simulink library "RCD2"  (R2025b)
settings: Solver=VariableStepAuto  StartTime=0.0  StopTime=10.0  RelTol=1e-3
libraries: simulink x73, etargetslib x4, $bdroot x2
(part 1 of 2)
settings Model: Creator=Eisenblaetter  LastModifiedBy=Scythe
settings OptimizationCC: ReuseModelBlockBuffer=off
settings RTWCC: GPUComputeCapability=3.5

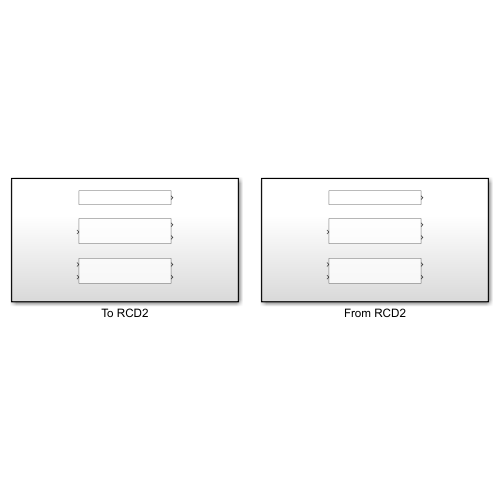
[thumbnail: Simulink's stored preview of the top-level diagram]
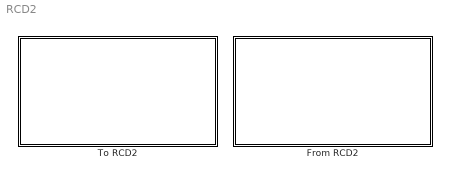
== system RCD2 ==
  From RCD2 : Subsystem
  To RCD2 : Subsystem

== system RCD2/From RCD2 ==
  RCD2 Actual Empty Bus : Subsystem
      mask help:
      | Create an empty RCD2 actual bus. All values are set to zero.<br><br>
      | The LED values are defined as follows:
      | <table style="background-color: #f8f8f8; border-style: solid; border-width: 1px; border-color: #ddd;" cellspacing="0" cellpadding ="2">
      | <tr style="background-color: #fff; text-align: left;"><th>Value</th><th>Description</th></tr>
      | <tr><td>0</td><td>LED off</td></tr>
      | <tr><td>1</td><td><span style="color: #f00;">RED</span> channel on, all others off</td></tr>
      | <tr><td>2</td><td><span style="color: #0f0;">GREEN</span> channel on, all others off</td></tr>
      | <tr><td>3</td><td><span style="color: #00f;">BLUE</span> channel on, all others off</td></tr>
      | </table>
      mask DialogControl DescGroupVar Prompt: RCD2 Actual - Empty Bus
      mask Display: disp('RCD2 Actual\nEmpty Bus');
  RCD2 Actual Pack : Subsystem  mask{idRCD=1}
      mask prompts: idRCD "ID of the RCD (0-255):"
      mask help:
      | Pack an RCD2 actual message to be sent from the RCD.<br><br>
      | The LED values are defined as follows:
      | <table style="background-color: #f8f8f8; border-style: solid; border-width: 1px; border-color: #ddd;" cellspacing="0" cellpadding ="2">
      | <tr style="background-color: #fff; text-align: left;"><th>Value</th><th>Description</th></tr>
      | <tr><td>0</td><td>LED off</td></tr>
      | <tr><td>1</td><td><span style="color: #f00;">RED</span> channel on, all others off</td></tr>
      | <tr><td>2</td><td><span style="color: #0f0;">GREEN</span> channel on, all others off</td></tr>
      | <tr><td>3</td><td><span style="color: #00f;">BLUE</span> channel on, all others off</td></tr>
      | </table>
      mask DialogControl DescGroupVar Prompt: RCD2 Actual - Pack
      mask Display:
      | id = get_param(gcb, 'idRCD');
      | disp(['RCD2 Actual\nPack\nID: ',id]);
  RCD2 Actual Unpack : Subsystem  mask{idRCD=1}
      mask prompts: idRCD "ID of the RCD (0-255):"
      mask help:
      | Pack an RCD2 actual message to be sent from the RCD.<br><br>
      | The LED values are defined as follows:
      | <table style="background-color: #f8f8f8; border-style: solid; border-width: 1px; border-color: #ddd;" cellspacing="0" cellpadding ="2">
      | <tr style="background-color: #fff; text-align: left;"><th>Value</th><th>Description</th></tr>
      | <tr><td>0</td><td>LED off</td></tr>
      | <tr><td>1</td><td><span style="color: #f00;">RED</span> channel on, all others off</td></tr>
      | <tr><td>2</td><td><span style="color: #0f0;">GREEN</span> channel on, all others off</td></tr>
      | <tr><td>3</td><td><span style="color: #00f;">BLUE</span> channel on, all others off</td></tr>
      | </table>
      mask DialogControl DescGroupVar Prompt: RCD2 Actual - Unpack
      mask Display:
      | id = get_param(gcb, 'idRCD');
      | disp(['RCD2 Actual\nUnpack\nID: ',id]);

== system RCD2/To RCD2 ==
  RCD2 Command Empty Bus : Subsystem
      mask help:
      | Create an empty RCD2 command bus. All values are set to zero and strings are empty.<br><br>
      | The LED values are defined as follows:
      | <table style="background-color: #f8f8f8; border-style: solid; border-width: 1px; border-color: #ddd;" cellspacing="0" cellpadding ="2">
      | <tr style="background-color: #fff; text-align: left;"><th>Value</th><th>Description</th></tr>
      | <tr><td>0</td><td>LED off</td></tr>
      | <tr><td>1</td><td><span style="color: #f00;">RED</span> channel on, all others off</td></tr>
      | <tr><td>2</td><td><span style="color: #0f0;">GREEN</span> channel on, all others off</td></tr>
      | <tr><td>3</td><td><span style="color: #00f;">BLUE</span> channel on, all others off</td></tr>
      | </table>
      mask DialogControl DescGroupVar Prompt: RCD2 Command - Empty Bus
      mask Display: disp('RCD2 Command\nEmpty Bus');
  RCD2 Command Pack : Subsystem  mask{idRCD=1}
      mask prompts: idRCD "ID of the RCD (0-255):"
      mask help:
      | Pack an RCD2 command message to be sent to the RCD.<br><br>
      | The LED values are defined as follows:
      | <table style="background-color: #f8f8f8; border-style: solid; border-width: 1px; border-color: #ddd;" cellspacing="0" cellpadding ="2">
      | <tr style="background-color: #fff; text-align: left;"><th>Value</th><th>Description</th></tr>
      | <tr><td>0</td><td>LED off</td></tr>
      | <tr><td>1</td><td><span style="color: #f00;">RED</span> channel on, all others off</td></tr>
      | <tr><td>2</td><td><span style="color: #0f0;">GREEN</span> channel on, all others off</td></tr>
      | <tr><td>3</td><td><span style="color: #00f;">BLUE</span> channel on, all others off</td></tr>
      | </table>
      mask DialogControl DescGroupVar Prompt: RCD2 Command - Pack
      mask Display:
      | id = get_param(gcb, 'idRCD');
      | disp(['RCD2 Command\nPack\nID: ',id]);
  RCD2 Command Unpack : Subsystem  mask{idRCD=1}
      mask prompts: idRCD "ID of the RCD (0-255):"
      mask help:
      | Unpack an RCD2 command message that has been sent to the RCD.<br><br>
      | The LED values are defined as follows:
      | <table style="background-color: #f8f8f8; border-style: solid; border-width: 1px; border-color: #ddd;" cellspacing="0" cellpadding ="2">
      | <tr style="background-color: #fff; text-align: left;"><th>Value</th><th>Description</th></tr>
      | <tr><td>0</td><td>LED off</td></tr>
      | <tr><td>1</td><td><span style="color: #f00;">RED</span> channel on, all others off</td></tr>
      | <tr><td>2</td><td><span style="color: #0f0;">GREEN</span> channel on, all others off</td></tr>
      | <tr><td>3</td><td><span style="color: #00f;">BLUE</span> channel on, all others off</td></tr>
      | </table>
      mask DialogControl DescGroupVar Prompt: RCD2 Command - Unpack
      mask Display:
      | id = get_param(gcb, 'idRCD');
      | disp(['RCD2 Command\nUnpack\nID: ',id]);

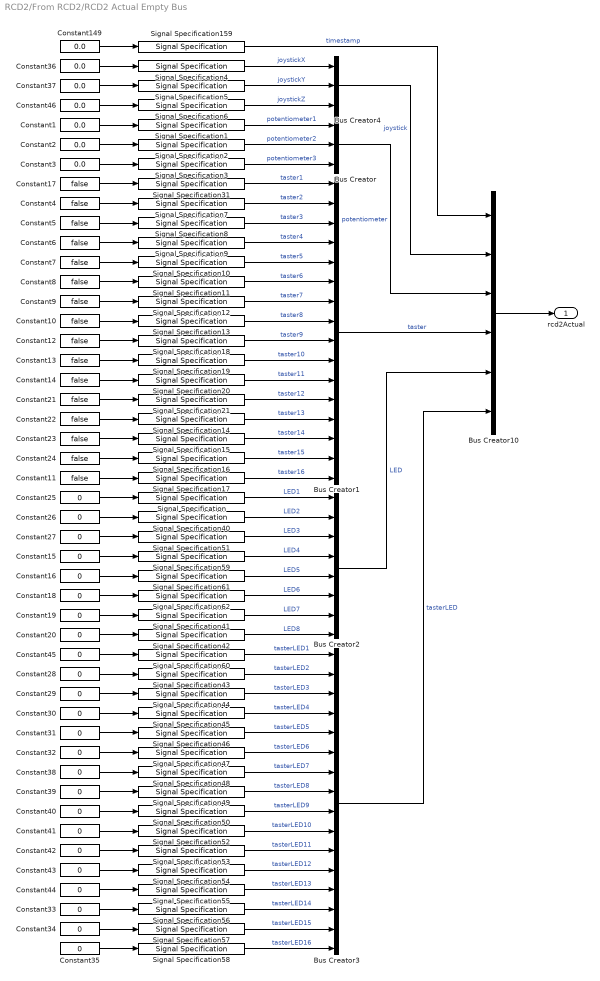
== system RCD2/From RCD2/RCD2 Actual Empty Bus ==
  Bus Creator : BusCreator  Inputs=3
  Bus Creator1 : BusCreator  Inputs=16
  Bus Creator10 : BusCreator  Inputs=6
  Bus Creator2 : BusCreator  Inputs=8
  Bus Creator3 : BusCreator  Inputs=16
  Bus Creator4 : BusCreator  Inputs=3
  Constant{1..3,36..37,46,149} (7 alike) : Constant  Value=0.0  OutDataTypeStr=double
  Constant{4..14,17,21..24} (16 alike) : Constant  Value=false  OutDataTypeStr=boolean
  Constant{15..16,18..20,25..35,38..45} (24 alike) : Constant  Value=0  OutDataTypeStr=uint8
  Signal Specification{,40..62} (24 alike) : SignalSpecification  OutDataTypeStr=uint8  Dimensions=1
  Signal Specification{1..6} (6 alike) : SignalSpecification  OutDataTypeStr=double  Dimensions=1
  Signal Specification{7..21,31} (16 alike) : SignalSpecification  OutDataTypeStr=boolean  Dimensions=1
  Signal Specification159 : SignalSpecification  OutDataTypeStr=double  Unit=s  Dimensions=1
  rcd2Actual : Outport
  wires:
  Bus Creator/1 -> Bus Creator10/3  "potentiometer"
  Signal Specification159/1 -> Bus Creator10/1  "timestamp"
  Bus Creator10/1 -> rcd2Actual/1
  Bus Creator1/1 -> Bus Creator10/4  "taster"
  Constant149/1 -> Signal Specification159/1
  Signal Specification53/1 -> Bus Creator3/11  "tasterLED11"
  Bus Creator2/1 -> Bus Creator10/5  "LED"
  Signal Specification55/1 -> Bus Creator3/13  "tasterLED13"
  Signal Specification43/1 -> Bus Creator3/2  "tasterLED2"
  Signal Specification50/1 -> Bus Creator3/9  "tasterLED9"
  Signal Specification51/1 -> Bus Creator2/3  "LED3"
  Signal Specification57/1 -> Bus Creator3/15  "tasterLED15"
  Signal Specification/1 -> Bus Creator2/1  "LED1"
  Signal Specification62/1 -> Bus Creator2/6  "LED6"
  Signal Specification59/1 -> Bus Creator2/4  "LED4"
  Bus Creator3/1 -> Bus Creator10/6  "tasterLED"
  Signal Specification49/1 -> Bus Creator3/8  "tasterLED8"
  Signal Specification44/1 -> Bus Creator3/3  "tasterLED3"
  Signal Specification40/1 -> Bus Creator2/2  "LED2"
  Signal Specification61/1 -> Bus Creator2/5  "LED5"
  Signal Specification45/1 -> Bus Creator3/4  "tasterLED4"
  Signal Specification42/1 -> Bus Creator2/8  "LED8"
  Signal Specification47/1 -> Bus Creator3/6  "tasterLED6"
  Signal Specification46/1 -> Bus Creator3/5  "tasterLED5"
  Signal Specification52/1 -> Bus Creator3/10  "tasterLED10"
  Signal Specification60/1 -> Bus Creator3/1  "tasterLED1"
  Signal Specification48/1 -> Bus Creator3/7  "tasterLED7"
  Signal Specification58/1 -> Bus Creator3/16  "tasterLED16"
  Signal Specification56/1 -> Bus Creator3/14  "tasterLED14"
  Signal Specification41/1 -> Bus Creator2/7  "LED7"
  Signal Specification54/1 -> Bus Creator3/12  "tasterLED12"
  Signal Specification21/1 -> Bus Creator1/12  "taster12"
  Signal Specification15/1 -> Bus Creator1/14  "taster14"
  Signal Specification17/1 -> Bus Creator1/16  "taster16"
  Constant17/1 -> Signal Specification31/1
  Signal Specification12/1 -> Bus Creator1/7  "taster7"
  Signal Specification31/1 -> Bus Creator1/1  "taster1"
  Signal Specification19/1 -> Bus Creator1/10  "taster10"
  Signal Specification10/1 -> Bus Creator1/5  "taster5"
  Signal Specification11/1 -> Bus Creator1/6  "taster6"
  Signal Specification9/1 -> Bus Creator1/4  "taster4"
  Signal Specification8/1 -> Bus Creator1/3  "taster3"
  Signal Specification13/1 -> Bus Creator1/8  "taster8"
  Signal Specification16/1 -> Bus Creator1/15  "taster15"
  Signal Specification18/1 -> Bus Creator1/9  "taster9"
  Signal Specification7/1 -> Bus Creator1/2  "taster2"
  Signal Specification14/1 -> Bus Creator1/13  "taster13"
  Signal Specification20/1 -> Bus Creator1/11  "taster11"
  Constant1/1 -> Signal Specification1/1
  Signal Specification1/1 -> Bus Creator/1  "potentiometer1"
  Constant2/1 -> Signal Specification2/1
  Signal Specification2/1 -> Bus Creator/2  "potentiometer2"
  Constant3/1 -> Signal Specification3/1
  Signal Specification3/1 -> Bus Creator/3  "potentiometer3"
  Constant27/1 -> Signal Specification51/1
  Constant15/1 -> Signal Specification59/1
  Constant16/1 -> Signal Specification61/1
  Constant20/1 -> Signal Specification42/1
  Constant19/1 -> Signal Specification41/1
  Constant18/1 -> Signal Specification62/1
  Constant25/1 -> Signal Specification/1
  Constant26/1 -> Signal Specification40/1
  Constant38/1 -> Signal Specification48/1
  Constant39/1 -> Signal Specification49/1
  Constant40/1 -> Signal Specification50/1
  Constant43/1 -> Signal Specification54/1
  Constant42/1 -> Signal Specification53/1
  Constant41/1 -> Signal Specification52/1
  Constant35/1 -> Signal Specification58/1
  Constant34/1 -> Signal Specification57/1
  Constant33/1 -> Signal Specification56/1
  Constant44/1 -> Signal Specification55/1
  Constant45/1 -> Signal Specification60/1
  Constant28/1 -> Signal Specification43/1
  Constant29/1 -> Signal Specification44/1
  Constant32/1 -> Signal Specification47/1
  Constant31/1 -> Signal Specification46/1
  Constant30/1 -> Signal Specification45/1
  Signal Specification6/1 -> Bus Creator4/3  "joystickZ"
  Constant46/1 -> Signal Specification6/1
  Signal Specification5/1 -> Bus Creator4/2  "joystickY"
  Constant37/1 -> Signal Specification5/1
  Signal Specification4/1 -> Bus Creator4/1  "joystickX"
  Constant36/1 -> Signal Specification4/1
  Bus Creator4/1 -> Bus Creator10/2  "joystick"
  Constant4/1 -> Signal Specification7/1
  Constant6/1 -> Signal Specification9/1
  Constant5/1 -> Signal Specification8/1
  Constant9/1 -> Signal Specification12/1
  Constant10/1 -> Signal Specification13/1
  Constant8/1 -> Signal Specification11/1
  Constant7/1 -> Signal Specification10/1
  Constant22/1 -> Signal Specification14/1
  Constant23/1 -> Signal Specification15/1
  Constant11/1 -> Signal Specification17/1
  Constant24/1 -> Signal Specification16/1
  Constant14/1 -> Signal Specification20/1
  Constant21/1 -> Signal Specification21/1
  Constant13/1 -> Signal Specification19/1
  Constant12/1 -> Signal Specification18/1

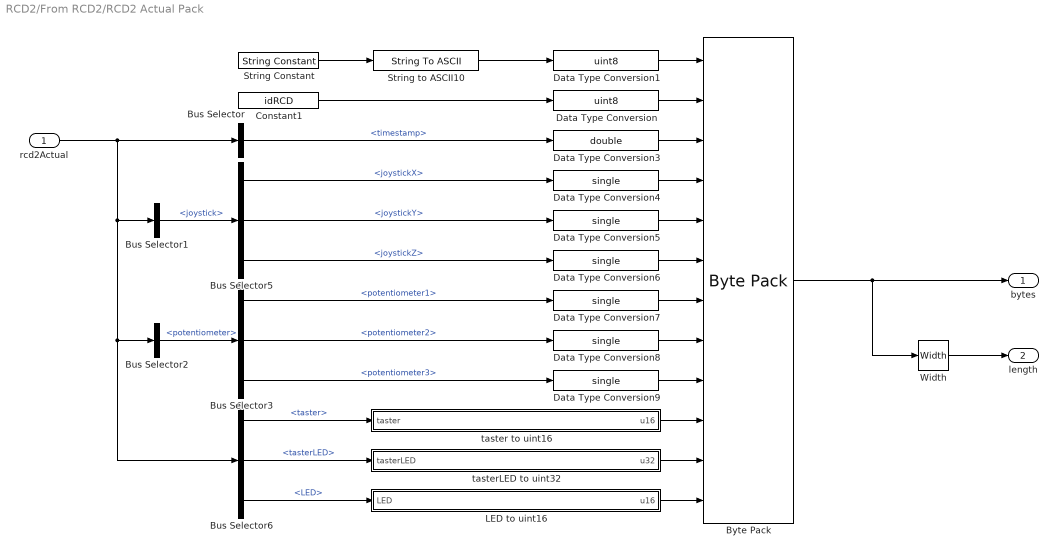
== system RCD2/From RCD2/RCD2 Actual Pack ==
  rcd2Actual : Inport
  Bus Selector : BusSelector  OutputSignals=timestamp
  Bus Selector1 : BusSelector  OutputSignals=joystick
  Bus Selector2 : BusSelector  OutputSignals=potentiometer
  Bus Selector3 : BusSelector  OutputSignals=potentiometer1,potentiometer2,potentiometer3
  Bus Selector5 : BusSelector  OutputSignals=joystickX,joystickY,joystickZ
  Bus Selector6 : BusSelector  OutputSignals=taster,tasterLED,LED
  Byte Pack : etargetslib/Byte Pack  datatypes={'uint8','uint8','double','single','single','single','single','single','single','uint16','uint32','uint16'}  byteAlign=1
  Constant1 : Constant  Value=idRCD  OutDataTypeStr=uint8
  Data Type Conversion : DataTypeConversion  OutDataTypeStr=uint8  SaturateOnIntegerOverflow=off  RndMeth=Floor
  Data Type Conversion1 : DataTypeConversion  OutDataTypeStr=uint8  SaturateOnIntegerOverflow=off  RndMeth=Floor
  Data Type Conversion3 : DataTypeConversion  OutDataTypeStr=double  SaturateOnIntegerOverflow=off  RndMeth=Floor
  Data Type Conversion{4..9} (6 alike) : DataTypeConversion  OutDataTypeStr=single  SaturateOnIntegerOverflow=off  RndMeth=Floor
  LED to uint16 : Subsystem
  String Constant : StringConstant  String="\"RCD2\""
  String to ASCII10 : StringToASCII  OutputVectorSize=4
  Width : Width  DataType=int32
  taster to uint16 : Subsystem
  tasterLED to uint32 : Subsystem
  bytes : Outport  OutDataTypeStr=uint8
  length : Outport  Port=2  OutDataTypeStr=int32  PortDimensions=1
  wires:
  Bus Selector5/1 -> Data Type Conversion4/1  "<joystickX>"
  Bus Selector5/2 -> Data Type Conversion5/1  "<joystickY>"
  Width/1 -> length/1
  Bus Selector5/3 -> Data Type Conversion6/1  "<joystickZ>"
  String Constant/1 -> String to ASCII10/1
  Constant1/1 -> Data Type Conversion/1
  String to ASCII10/1 -> Data Type Conversion1/1
  Bus Selector/1 -> Data Type Conversion3/1  "<timestamp>"
  Byte Pack/1 -> Width/1, bytes/1
  Bus Selector1/1 -> Bus Selector5/1  "<joystick>"
  Bus Selector2/1 -> Bus Selector3/1  "<potentiometer>"
  Bus Selector3/3 -> Data Type Conversion9/1  "<potentiometer3>"
  Bus Selector3/2 -> Data Type Conversion8/1  "<potentiometer2>"
  Bus Selector3/1 -> Data Type Conversion7/1  "<potentiometer1>"
  rcd2Actual/1 -> Bus Selector6/1, Bus Selector2/1, Bus Selector1/1, Bus Selector/1
  Bus Selector6/1 -> taster to uint16/1("taster ")  "<taster>"
  Bus Selector6/2 -> tasterLED to uint32/1("tasterLED ")  "<tasterLED>"
  Bus Selector6/3 -> LED to uint16/1("LED ")  "<LED>"
  Data Type Conversion6/1 -> Byte Pack/6
  Data Type Conversion7/1 -> Byte Pack/7
  Data Type Conversion8/1 -> Byte Pack/8
  Data Type Conversion9/1 -> Byte Pack/9
  taster to uint16/1(u16) -> Byte Pack/10
  tasterLED to uint32/1(u32) -> Byte Pack/11
  LED to uint16/1(u16) -> Byte Pack/12
  Data Type Conversion4/1 -> Byte Pack/4
  Data Type Conversion5/1 -> Byte Pack/5
  Data Type Conversion3/1 -> Byte Pack/3
  Data Type Conversion/1 -> Byte Pack/2
  Data Type Conversion1/1 -> Byte Pack/1

== system RCD2/From RCD2/RCD2 Actual Unpack ==
  bytes : Inport  OutDataTypeStr=uint8
  length : Inport  Port=2  OutDataTypeStr=int32  PortDimensions=1
  AND : Logic  AllPortsSameDT=off  OutDataTypeStr=boolean
  AND1 : Logic  AllPortsSameDT=off  OutDataTypeStr=boolean
  Check Message Size : simulink/Logic and Bit Operations/Compare To Constant  relop===  const=int32(45)  OutDataTypeStr=boolean
  Relational Operator : RelationalOperator  Operator=<=  OutDataTypeStr=boolean  RndMeth=Simplest  InputSameDT=off
  Unpack Message : Subsystem  TreatAsAtomicUnit=on
  Width : Width  DataType=int32
  success : Outport  OutDataTypeStr=boolean  PortDimensions=1
  rcd2Actual : Outport  Port=2
  wires:
  Unpack Message/1(success) -> AND/2
  Unpack Message/2(busRCDActual) -> rcd2Actual/1
  AND1/1 -> Unpack Message/Enable, AND/1
  AND/1 -> success/1
  Width/1 -> Relational Operator/2
  length/1 -> Relational Operator/1, Check Message Size/1
  Relational Operator/1 -> AND1/2
  bytes/1 -> Width/1, Unpack Message/1(bytes)
  Check Message Size/1 -> AND1/1

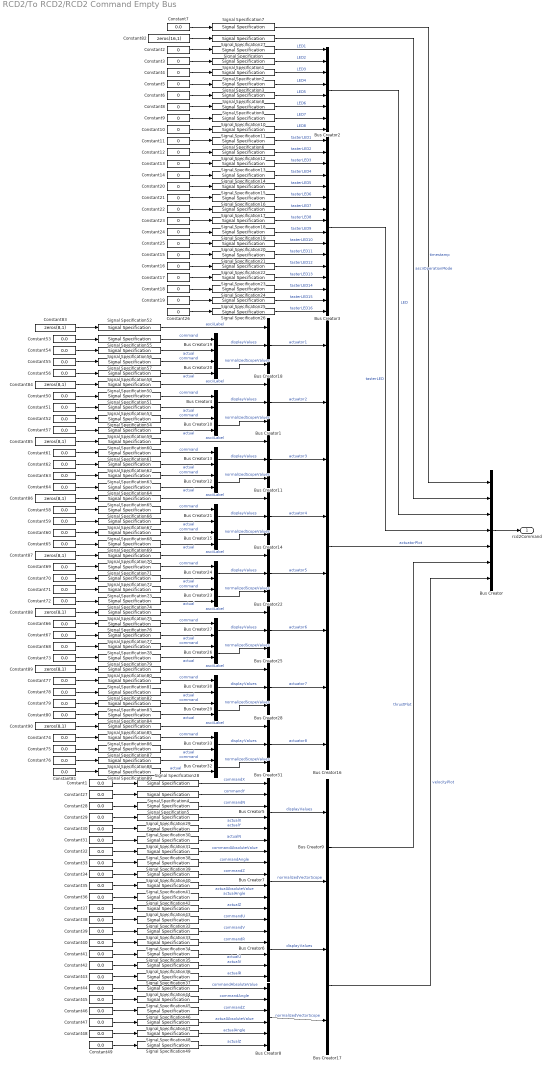
== system RCD2/To RCD2/RCD2 Command Empty Bus ==
  Bus Creator : BusCreator  Inputs=7
  Bus Creator{1,11,14,18,22,25,28,31} (8 alike) : BusCreator  Inputs=3
  Bus Creator{4,9..10,12..13,15,17,19..21,23..24,26..27,29..30,32..33} (18 alike) : BusCreator  Inputs=2
  Bus Creator16 : BusCreator  Inputs=8
  Bus Creator2 : BusCreator  Inputs=8
  Bus Creator3 : BusCreator  Inputs=16
  Bus Creator{5..8} (4 alike) : BusCreator  Inputs=6
  Constant{1,7,27..81} (57 alike) : Constant  Value=0.0  OutDataTypeStr=double
  Constant{2..6,8..26} (24 alike) : Constant  Value=0  OutDataTypeStr=uint8
  Constant82 : Constant  Value=zeros(16,1)  OutDataTypeStr=uint8
  Constant{83..90} (8 alike) : Constant  Value=zeros(8,1)  OutDataTypeStr=uint8
  Signal Specification{,1..3,6,8..26} (24 alike) : SignalSpecification  OutDataTypeStr=uint8  Dimensions=1
  Signal Specification27 : SignalSpecification  OutDataTypeStr=uint8  Dimensions=16
  Signal Specification{4..5,28..49,51,53..59,61..64,66..69,71..74,76..79,81..84,86..89} (56 alike) : SignalSpecification  OutDataTypeStr=double  Dimensions=1
  Signal Specification{50,52,60,65,70,75,80,85} (8 alike) : SignalSpecification  OutDataTypeStr=uint8  Dimensions=8
  Signal Specification7 : SignalSpecification  OutDataTypeStr=double  Unit=s  Dimensions=1
  rcd2Command : Outport
  wires:
  Bus Creator/1 -> rcd2Command/1
  Signal Specification22/1 -> Bus Creator3/12  "tasterLED12"
  Signal Specification5/1 -> Bus Creator5/3  "commandN"
  Constant39/1 -> Signal Specification33/1
  Constant29/1 -> Signal Specification29/1
  Bus Creator17/1 -> Bus Creator/7  "velocityPlot"
  Signal Specification23/1 -> Bus Creator3/13  "tasterLED13"
  Signal Specification2/1 -> Bus Creator2/3  "LED3"
  Signal Specification26/1 -> Bus Creator3/16  "tasterLED16"
  Constant82/1 -> Signal Specification27/1
  Constant15/1 -> Signal Specification21/1
  Constant7/1 -> Signal Specification7/1
  Constant2/1 -> Signal Specification/1
  Constant14/1 -> Signal Specification14/1
  Signal Specification16/1 -> Bus Creator3/6  "tasterLED6"
  Constant42/1 -> Signal Specification36/1
  Constant25/1 -> Signal Specification20/1
  Signal Specification30/1 -> Bus Creator5/5  "actualY"
  Bus Creator3/1 -> Bus Creator/4  "tasterLED"
  Bus Creator16/1 -> Bus Creator/5  "actuatorPlot"
  Signal Specification11/1 -> Bus Creator2/8  "LED8"
  Signal Specification17/1 -> Bus Creator3/7  "tasterLED7"
  Signal Specification29/1 -> Bus Creator5/4  "actualX"
  Constant28/1 -> Signal Specification5/1
  Constant12/1 -> Signal Specification12/1
  Constant31/1 -> Signal Specification31/1
  Signal Specification39/1 -> Bus Creator7/2  "commandAngle"
  Signal Specification10/1 -> Bus Creator2/7  "LED7"
  Signal Specification31/1 -> Bus Creator5/6  "actualN"
  Signal Specification1/1 -> Bus Creator2/2  "LED2"
  Signal Specification9/1 -> Bus Creator2/6  "LED6"
  Constant8/1 -> Signal Specification9/1
  Signal Specification4/1 -> Bus Creator5/2  "commandY"
  Constant17/1 -> Signal Specification23/1
  Bus Creator9/1 -> Bus Creator/6  "thrustPlot"
  Constant30/1 -> Signal Specification30/1
  Constant1/1 -> Signal Specification28/1
  Constant18/1 -> Signal Specification24/1
  Signal Specification35/1 -> Bus Creator6/4  "actualU"
  Constant5/1 -> Signal Specification3/1
  Signal Specification36/1 -> Bus Creator6/5  "actualV"
  Constant32/1 -> Signal Specification38/1
  Signal Specification14/1 -> Bus Creator3/4  "tasterLED4"
  Signal Specification21/1 -> Bus Creator3/11  "tasterLED11"
  Signal Specification42/1 -> Bus Creator7/5  "actualAngle"
  Signal Specification13/1 -> Bus Creator3/3  "tasterLED3"
  Bus Creator2/1 -> Bus Creator/3  "LED"
  Constant41/1 -> Signal Specification35/1
  Constant40/1 -> Signal Specification34/1
  Constant34/1 -> Signal Specification40/1
  Constant38/1 -> Signal Specification32/1
  Signal Specification34/1 -> Bus Creator6/3  "commandR"
  Constant27/1 -> Signal Specification4/1
  Signal Specification32/1 -> Bus Creator6/1  "commandU"
  Signal Specification28/1 -> Bus Creator5/1  "commandX"
  Signal Specification33/1 -> Bus Creator6/2  "commandV"
  Signal Specification40/1 -> Bus Creator7/3  "commandZ"
  Signal Specification/1 -> Bus Creator2/1  "LED1"
  Constant43/1 -> Signal Specification37/1
  Constant26/1 -> Signal Specification26/1
  Constant37/1 -> Signal Specification43/1
  Constant35/1 -> Signal Specification41/1
  Signal Specification20/1 -> Bus Creator3/10  "tasterLED10"
  Signal Specification38/1 -> Bus Creator7/1  "commandAbsoluteValue"
  Constant3/1 -> Signal Specification1/1
  Constant36/1 -> Signal Specification42/1
  Signal Specification3/1 -> Bus Creator2/4  "LED4"
  Signal Specification24/1 -> Bus Creator3/14  "tasterLED14"
  Constant16/1 -> Signal Specification22/1
  Constant19/1 -> Signal Specification25/1
  Signal Specification12/1 -> Bus Creator3/2  "tasterLED2"
  Constant20/1 -> Signal Specification15/1
  Constant11/1 -> Signal Specification6/1
  Constant9/1 -> Signal Specification10/1
  Signal Specification43/1 -> Bus Creator7/6  "actualZ"
  Constant10/1 -> Signal Specification11/1
  Signal Specification19/1 -> Bus Creator3/9  "tasterLED9"
  Constant6/1 -> Signal Specification8/1
  Constant21/1 -> Signal Specification16/1
  Signal Specification15/1 -> Bus Creator3/5  "tasterLED5"
  Signal Specification25/1 -> Bus Creator3/15  "tasterLED15"
  Constant33/1 -> Signal Specification39/1
  Constant13/1 -> Signal Specification13/1
  Signal Specification37/1 -> Bus Creator6/6  "actualR"
  Signal Specification18/1 -> Bus Creator3/8  "tasterLED8"
  Signal Specification8/1 -> Bus Creator2/5  "LED5"
  Signal Specification41/1 -> Bus Creator7/4  "actualAbsoluteValue"
  Constant23/1 -> Signal Specification18/1
  Constant24/1 -> Signal Specification19/1
  Constant4/1 -> Signal Specification2/1
  Signal Specification6/1 -> Bus Creator3/1  "tasterLED1"
  Signal Specification7/1 -> Bus Creator/1  "timestamp"
  Constant22/1 -> Signal Specification17/1
  Signal Specification27/1 -> Bus Creator/2  "asciiOperationMode"
  Signal Specification47/1 -> Bus Creator8/4  "actualAbsoluteValue"
  Constant45/1 -> Signal Specification45/1
  Signal Specification49/1 -> Bus Creator8/6  "actualZ"
  Constant48/1 -> Signal Specification48/1
  Signal Specification44/1 -> Bus Creator8/1  "commandAbsoluteValue"
  Constant47/1 -> Signal Specification47/1
  Constant49/1 -> Signal Specification49/1
  Signal Specification46/1 -> Bus Creator8/3  "commandZ"
  Constant46/1 -> Signal Specification46/1
  Signal Specification48/1 -> Bus Creator8/5  "actualAngle"
  Constant44/1 -> Signal Specification44/1
  Signal Specification45/1 -> Bus Creator8/2  "commandAngle"
  Bus Creator11/1 -> Bus Creator16/3  "actuator3"
  Bus Creator14/1 -> Bus Creator16/4  "actuator4"
  Bus Creator1/1 -> Bus Creator16/2  "actuator2"
  Bus Creator22/1 -> Bus Creator16/5  "actuator5"
  Bus Creator18/1 -> Bus Creator16/1  "actuator1"
  Bus Creator25/1 -> Bus Creator16/6  "actuator6"
  Bus Creator28/1 -> Bus Creator16/7  "actuator7"
  Bus Creator31/1 -> Bus Creator16/8  "actuator8"
  Bus Creator5/1 -> Bus Creator9/1  "displayValues"
  Bus Creator7/1 -> Bus Creator9/2  "normalizedVectorScope"
  Bus Creator6/1 -> Bus Creator17/1  "displayValues"
  Bus Creator8/1 -> Bus Creator17/2  "normalizedVectorScope"
  Constant54/1 -> Signal Specification56/1
  Constant53/1 -> Signal Specification55/1
  Signal Specification56/1 -> Bus Creator19/2  "actual"
  Signal Specification52/1 -> Bus Creator18/1  "asciiLabel"
  Constant83/1 -> Signal Specification52/1
  Signal Specification55/1 -> Bus Creator19/1  "command"
  Bus Creator19/1 -> Bus Creator18/2  "displayValues"
  Bus Creator20/1 -> Bus Creator18/3  "normalizedScopeValues"
  Signal Specification57/1 -> Bus Creator20/1  "command"
  Signal Specification58/1 -> Bus Creator20/2  "actual"
  Constant55/1 -> Signal Specification57/1
  Constant56/1 -> Signal Specification58/1
  Constant57/1 -> Signal Specification59/1
  Constant52/1 -> Signal Specification54/1
  Signal Specification59/1 -> Bus Creator10/2  "actual"
  Signal Specification54/1 -> Bus Creator10/1  "command"
  Bus Creator10/1 -> Bus Creator1/3  "normalizedScopeValues"
  Bus Creator4/1 -> Bus Creator1/2  "displayValues"
  Signal Specification51/1 -> Bus Creator4/1  "command"
  Signal Specification53/1 -> Bus Creator4/2  "actual"
  Constant50/1 -> Signal Specification51/1
  Constant51/1 -> Signal Specification53/1
  Constant62/1 -> Signal Specification62/1
  Constant61/1 -> Signal Specification61/1
  Signal Specification62/1 -> Bus Creator13/2  "actual"
  Signal Specification61/1 -> Bus Creator13/1  "command"
  Bus Creator13/1 -> Bus Creator11/2  "displayValues"
  Bus Creator12/1 -> Bus Creator11/3  "normalizedScopeValues"
  Signal Specification63/1 -> Bus Creator12/1  "command"
  Signal Specification64/1 -> Bus Creator12/2  "actual"
  Constant63/1 -> Signal Specification63/1
  Constant64/1 -> Signal Specification64/1
  Constant65/1 -> Signal Specification69/1
  Constant60/1 -> Signal Specification68/1
  Signal Specification69/1 -> Bus Creator15/2  "actual"
  Signal Specification68/1 -> Bus Creator15/1  "command"
  Bus Creator15/1 -> Bus Creator14/3  "normalizedScopeValues"
  Bus Creator21/1 -> Bus Creator14/2  "displayValues"
  Signal Specification66/1 -> Bus Creator21/1  "command"
  Signal Specification67/1 -> Bus Creator21/2  "actual"
  Constant58/1 -> Signal Specification66/1
  Constant59/1 -> Signal Specification67/1
  Constant70/1 -> Signal Specification72/1
  Constant69/1 -> Signal Specification71/1
  Signal Specification72/1 -> Bus Creator24/2  "actual"
  Signal Specification71/1 -> Bus Creator24/1  "command"
  Bus Creator24/1 -> Bus Creator22/2  "displayValues"
  Bus Creator23/1 -> Bus Creator22/3  "normalizedScopeValues"
  Signal Specification73/1 -> Bus Creator23/1  "command"
  Signal Specification74/1 -> Bus Creator23/2  "actual"
  Constant71/1 -> Signal Specification73/1
  Constant72/1 -> Signal Specification74/1
  Constant73/1 -> Signal Specification79/1
  Constant68/1 -> Signal Specification78/1
  Signal Specification79/1 -> Bus Creator26/2  "actual"
  Signal Specification78/1 -> Bus Creator26/1  "command"
  Bus Creator26/1 -> Bus Creator25/3  "normalizedScopeValues"
  Bus Creator27/1 -> Bus Creator25/2  "displayValues"
  Signal Specification76/1 -> Bus Creator27/1  "command"
  Signal Specification77/1 -> Bus Creator27/2  "actual"
  Constant66/1 -> Signal Specification76/1
  Constant67/1 -> Signal Specification77/1
  Constant78/1 -> Signal Specification82/1
  Constant77/1 -> Signal Specification81/1
  Signal Specification82/1 -> Bus Creator30/2  "actual"
  Signal Specification81/1 -> Bus Creator30/1  "command"
  Bus Creator30/1 -> Bus Creator28/2  "displayValues"
  Bus Creator29/1 -> Bus Creator28/3  "normalizedScopeValues"
  Signal Specification83/1 -> Bus Creator29/1  "command"
  Signal Specification84/1 -> Bus Creator29/2  "actual"
  Constant79/1 -> Signal Specification83/1
  Constant80/1 -> Signal Specification84/1
  Constant81/1 -> Signal Specification89/1
  Constant76/1 -> Signal Specification88/1
  Signal Specification89/1 -> Bus Creator32/2  "actual"
  Signal Specification88/1 -> Bus Creator32/1  "command"
  Bus Creator32/1 -> Bus Creator31/3  "normalizedScopeValues"
  Bus Creator33/1 -> Bus Creator31/2  "displayValues"
  Signal Specification86/1 -> Bus Creator33/1  "command"
  Signal Specification87/1 -> Bus Creator33/2  "actual"
  Constant74/1 -> Signal Specification86/1
  Constant75/1 -> Signal Specification87/1
  Signal Specification50/1 -> Bus Creator1/1  "asciiLabel"
  Signal Specification60/1 -> Bus Creator11/1  "asciiLabel"
  Signal Specification65/1 -> Bus Creator14/1  "asciiLabel"
  Signal Specification70/1 -> Bus Creator22/1  "asciiLabel"
  Signal Specification75/1 -> Bus Creator25/1  "asciiLabel"
  Signal Specification80/1 -> Bus Creator28/1  "asciiLabel"
  Signal Specification85/1 -> Bus Creator31/1  "asciiLabel"
  Constant84/1 -> Signal Specification50/1
  Constant85/1 -> Signal Specification60/1
  Constant86/1 -> Signal Specification65/1
  Constant87/1 -> Signal Specification70/1
  Constant88/1 -> Signal Specification75/1
  Constant89/1 -> Signal Specification80/1
  Constant90/1 -> Signal Specification85/1

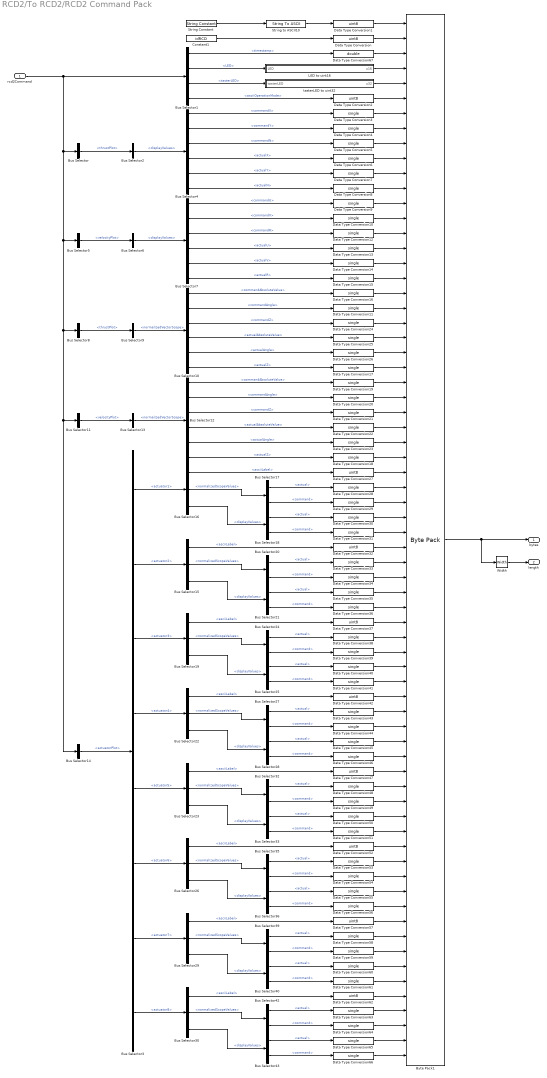
== system RCD2/To RCD2/RCD2 Command Pack ==
  rcd2Command : Inport
  Bus Selector : BusSelector  OutputSignals=thrustPlot
  Bus Selector1 : BusSelector  OutputSignals=timestamp,LED,tasterLED,asciiOperationMode
  Bus Selector10 : BusSelector  OutputSignals=commandAbsoluteValue,commandAngle,commandZ,actualAbsoluteValue,actualAngle,actualZ
  Bus Selector11 : BusSelector  OutputSignals=velocityPlot
  Bus Selector12 : BusSelector  OutputSignals=commandAbsoluteValue,commandAngle,commandZ,actualAbsoluteValue,actualAngle,actualZ
  Bus Selector13 : BusSelector  OutputSignals=normalizedVectorScope
  Bus Selector14 : BusSelector  OutputSignals=actuatorPlot
  Bus Selector{15..16,19,22..23,26,29..30} (8 alike) : BusSelector  OutputSignals=asciiLabel,normalizedScopeValues,displayValues
  Bus Selector{17..18,20..21,24..25,27..28,32..33,35..36,39..40,42..43} (16 alike) : BusSelector  OutputSignals=actual,command
  Bus Selector2 : BusSelector  OutputSignals=displayValues
  Bus Selector3 : BusSelector  OutputSignals=actuator1,actuator2,actuator3,actuator4,actuator5,actuator6,actuator7,actuator8
  Bus Selector4 : BusSelector  OutputSignals=commandX,commandY,commandN,actualX,actualY,actualN
  Bus Selector5 : BusSelector  OutputSignals=velocityPlot
  Bus Selector6 : BusSelector  OutputSignals=displayValues
  Bus Selector7 : BusSelector  OutputSignals=commandU,commandV,commandR,actualU,actualV,actualR
  Bus Selector8 : BusSelector  OutputSignals=thrustPlot
  Bus Selector9 : BusSelector  OutputSignals=normalizedVectorScope
  Byte Pack1 : etargetslib/Byte Pack  datatypes={'uint8', 'uint8', 'double', 'uint16','uint32','uint8','single','single','single','single','single','single','single','single','single','single','single','single','single','single','single','single','single','single','single','single','single','single','single','single','uint8','single','single','single','single','uint8','single','single','single','single','uint8','single','single','single','single','uint8','single','single','single','single','uint8','single','single','single','single','uint8','single','single','single','single','uint8','single','single','single','single','uint8','single','single','single','single'}  byteAlign=1
  Constant1 : Constant  Value=idRCD  OutDataTypeStr=uint8
  Data Type Conversion{,1..2,27,32,37,42,47,52,57,62} (11 alike) : DataTypeConversion  OutDataTypeStr=uint8  SaturateOnIntegerOverflow=off  RndMeth=Floor
  Data Type Conversion{3..26,28..31,33..36,38..41,43..46,48..51,53..56,58..61,63..66} (56 alike) : DataTypeConversion  OutDataTypeStr=single  SaturateOnIntegerOverflow=off  RndMeth=Floor
  Data Type Conversion67 : DataTypeConversion  OutDataTypeStr=double  SaturateOnIntegerOverflow=off  RndMeth=Floor
  LED to uint16 : Subsystem
  String Constant : StringConstant  String="\"RCD2\""
  String to ASCII10 : StringToASCII  OutputVectorSize=4
  Width : Width  DataType=int32
  tasterLED to uint32 : Subsystem
  bytes : Outport  OutDataTypeStr=uint8
  length : Outport  Port=2  OutDataTypeStr=int32  PortDimensions=1
  wires:
  Bus Selector1/3 -> tasterLED to uint32/1("tasterLED ")  "<tasterLED>"
  String to ASCII10/1 -> Data Type Conversion1/1
  Bus Selector1/2 -> LED to uint16/1("LED ")  "<LED>"
  Bus Selector1/4 -> Data Type Conversion2/1  "<asciiOperationMode>"
  String Constant/1 -> String to ASCII10/1
  tasterLED to uint32/1(u32) -> Byte Pack1/5
  Bus Selector1/1 -> Data Type Conversion67/1  "<timestamp>"
  LED to uint16/1(u16) -> Byte Pack1/4
  Data Type Conversion/1 -> Byte Pack1/2
  Byte Pack1/1 -> Width/1, bytes/1
  Width/1 -> length/1
  Constant1/1 -> Data Type Conversion/1
  Data Type Conversion1/1 -> Byte Pack1/1
  Data Type Conversion2/1 -> Byte Pack1/6
  Data Type Conversion3/1 -> Byte Pack1/7
  Data Type Conversion4/1 -> Byte Pack1/8
  Data Type Conversion5/1 -> Byte Pack1/9
  Data Type Conversion6/1 -> Byte Pack1/10
  Data Type Conversion7/1 -> Byte Pack1/11
  Data Type Conversion8/1 -> Byte Pack1/12
  Data Type Conversion9/1 -> Byte Pack1/13
  Data Type Conversion10/1 -> Byte Pack1/14
  Data Type Conversion12/1 -> Byte Pack1/15
  Data Type Conversion13/1 -> Byte Pack1/16
  Data Type Conversion14/1 -> Byte Pack1/17
  Data Type Conversion15/1 -> Byte Pack1/18
  Data Type Conversion16/1 -> Byte Pack1/19
  Data Type Conversion11/1 -> Byte Pack1/20
  Data Type Conversion24/1 -> Byte Pack1/21
  Data Type Conversion25/1 -> Byte Pack1/22
  Data Type Conversion26/1 -> Byte Pack1/23
  Data Type Conversion17/1 -> Byte Pack1/24
  Data Type Conversion19/1 -> Byte Pack1/25
  Data Type Conversion20/1 -> Byte Pack1/26
  Data Type Conversion21/1 -> Byte Pack1/27
  Data Type Conversion22/1 -> Byte Pack1/28
  Data Type Conversion23/1 -> Byte Pack1/29
  Data Type Conversion18/1 -> Byte Pack1/30
  Bus Selector/1 -> Bus Selector2/1  "<thrustPlot>"
  Bus Selector2/1 -> Bus Selector4/1  "<displayValues>"
  Bus Selector4/1 -> Data Type Conversion3/1  "<commandX>"
  Bus Selector4/2 -> Data Type Conversion4/1  "<commandY>"
  Bus Selector4/3 -> Data Type Conversion5/1  "<commandN>"
  Bus Selector4/4 -> Data Type Conversion6/1  "<actualX>"
  Bus Selector4/5 -> Data Type Conversion7/1  "<actualY>"
  Bus Selector4/6 -> Data Type Conversion8/1  "<actualN>"
  Bus Selector7/6 -> Data Type Conversion15/1  "<actualR>"
  Bus Selector7/5 -> Data Type Conversion14/1  "<actualV>"
  Bus Selector7/4 -> Data Type Conversion13/1  "<actualU>"
  Bus Selector7/3 -> Data Type Conversion12/1  "<commandR>"
  Bus Selector7/2 -> Data Type Conversion10/1  "<commandV>"
  Bus Selector7/1 -> Data Type Conversion9/1  "<commandU>"
  Bus Selector6/1 -> Bus Selector7/1  "<displayValues>"
  Bus Selector5/1 -> Bus Selector6/1  "<velocityPlot>"
  Bus Selector8/1 -> Bus Selector9/1  "<thrustPlot>"
  Bus Selector9/1 -> Bus Selector10/1  "<normalizedVectorScope>"
  Bus Selector10/1 -> Data Type Conversion16/1  "<commandAbsoluteValue>"
  Bus Selector10/2 -> Data Type Conversion11/1  "<commandAngle>"
  Bus Selector10/3 -> Data Type Conversion24/1  "<commandZ>"
  Bus Selector10/4 -> Data Type Conversion25/1  "<actualAbsoluteValue>"
  Bus Selector10/5 -> Data Type Conversion26/1  "<actualAngle>"
  Bus Selector10/6 -> Data Type Conversion17/1  "<actualZ>"
  Bus Selector12/6 -> Data Type Conversion18/1  "<actualZ>"
  Bus Selector12/5 -> Data Type Conversion23/1  "<actualAngle>"
  Bus Selector12/4 -> Data Type Conversion22/1  "<actualAbsoluteValue>"
  Bus Selector12/3 -> Data Type Conversion21/1  "<commandZ>"
  Bus Selector12/2 -> Data Type Conversion20/1  "<commandAngle>"
  Bus Selector12/1 -> Data Type Conversion19/1  "<commandAbsoluteValue>"
  Bus Selector13/1 -> Bus Selector12/1  "<normalizedVectorScope>"
  Bus Selector11/1 -> Bus Selector13/1  "<velocityPlot>"
  rcd2Command/1 -> Bus Selector14/1, Bus Selector11/1, Bus Selector8/1, Bus Selector5/1, Bus Selector/1, Bus Selector1/1
  Data Type Conversion27/1 -> Byte Pack1/31
  Bus Selector16/1 -> Data Type Conversion27/1  "<asciiLabel>"
  Bus Selector16/2 -> Bus Selector17/1  "<normalizedScopeValues>"
  Data Type Conversion28/1 -> Byte Pack1/32
  Data Type Conversion29/1 -> Byte Pack1/33
  Bus Selector17/1 -> Data Type Conversion28/1  "<actual>"
  Bus Selector17/2 -> Data Type Conversion29/1  "<command>"
  Bus Selector18/2 -> Data Type Conversion31/1  "<command>"
  Bus Selector18/1 -> Data Type Conversion30/1  "<actual>"
  Bus Selector16/3 -> Bus Selector18/1  "<displayValues>"
  Data Type Conversion30/1 -> Byte Pack1/34
  Data Type Conversion31/1 -> Byte Pack1/35
  Data Type Conversion36/1 -> Byte Pack1/40
  Data Type Conversion35/1 -> Byte Pack1/39
  Bus Selector15/3 -> Bus Selector21/1  "<displayValues>"
  Bus Selector21/1 -> Data Type Conversion35/1  "<actual>"
  Bus Selector21/2 -> Data Type Conversion36/1  "<command>"
  Bus Selector20/2 -> Data Type Conversion34/1  "<command>"
  Bus Selector20/1 -> Data Type Conversion33/1  "<actual>"
  Data Type Conversion34/1 -> Byte Pack1/38
  Data Type Conversion33/1 -> Byte Pack1/37
  Bus Selector15/2 -> Bus Selector20/1  "<normalizedScopeValues>"
  Bus Selector15/1 -> Data Type Conversion32/1  "<asciiLabel>"
  Data Type Conversion32/1 -> Byte Pack1/36
  Data Type Conversion42/1 -> Byte Pack1/46
  Bus Selector22/1 -> Data Type Conversion42/1  "<asciiLabel>"
  Bus Selector22/2 -> Bus Selector27/1  "<normalizedScopeValues>"
  Data Type Conversion43/1 -> Byte Pack1/47
  Data Type Conversion44/1 -> Byte Pack1/48
  Bus Selector27/1 -> Data Type Conversion43/1  "<actual>"
  Bus Selector27/2 -> Data Type Conversion44/1  "<command>"
  Bus Selector28/2 -> Data Type Conversion46/1  "<command>"
  Bus Selector28/1 -> Data Type Conversion45/1  "<actual>"
  Bus Selector22/3 -> Bus Selector28/1  "<displayValues>"
  Data Type Conversion45/1 -> Byte Pack1/49
  Data Type Conversion46/1 -> Byte Pack1/50
  Data Type Conversion41/1 -> Byte Pack1/45
  Data Type Conversion40/1 -> Byte Pack1/44
  Bus Selector19/3 -> Bus Selector25/1  "<displayValues>"
  Bus Selector25/1 -> Data Type Conversion40/1  "<actual>"
  Bus Selector25/2 -> Data Type Conversion41/1  "<command>"
  Bus Selector24/2 -> Data Type Conversion39/1  "<command>"
  Bus Selector24/1 -> Data Type Conversion38/1  "<actual>"
  Data Type Conversion39/1 -> Byte Pack1/43
  Data Type Conversion38/1 -> Byte Pack1/42
  Bus Selector19/2 -> Bus Selector24/1  "<normalizedScopeValues>"
  Bus Selector19/1 -> Data Type Conversion37/1  "<asciiLabel>"
  Data Type Conversion37/1 -> Byte Pack1/41
  Data Type Conversion57/1 -> Byte Pack1/61
  Bus Selector29/1 -> Data Type Conversion57/1  "<asciiLabel>"
  Bus Selector29/2 -> Bus Selector39/1  "<normalizedScopeValues>"
  Data Type Conversion58/1 -> Byte Pack1/62
  Data Type Conversion59/1 -> Byte Pack1/63
  Bus Selector39/1 -> Data Type Conversion58/1  "<actual>"
  Bus Selector39/2 -> Data Type Conversion59/1  "<command>"
  Bus Selector40/2 -> Data Type Conversion61/1  "<command>"
  Bus Selector40/1 -> Data Type Conversion60/1  "<actual>"
  Bus Selector29/3 -> Bus Selector40/1  "<displayValues>"
  Data Type Conversion60/1 -> Byte Pack1/64
  Data Type Conversion61/1 -> Byte Pack1/65
  Data Type Conversion66/1 -> Byte Pack1/70
  Data Type Conversion65/1 -> Byte Pack1/69
  Bus Selector30/3 -> Bus Selector43/1  "<displayValues>"
  Bus Selector43/1 -> Data Type Conversion65/1  "<actual>"
  Bus Selector43/2 -> Data Type Conversion66/1  "<command>"
  Bus Selector42/2 -> Data Type Conversion64/1  "<command>"
  Bus Selector42/1 -> Data Type Conversion63/1  "<actual>"
  Data Type Conversion64/1 -> Byte Pack1/68
  Data Type Conversion63/1 -> Byte Pack1/67
  Bus Selector30/2 -> Bus Selector42/1  "<normalizedScopeValues>"
  Bus Selector30/1 -> Data Type Conversion62/1  "<asciiLabel>"
  Data Type Conversion62/1 -> Byte Pack1/66
  Data Type Conversion52/1 -> Byte Pack1/56
  Bus Selector26/1 -> Data Type Conversion52/1  "<asciiLabel>"
  Bus Selector26/2 -> Bus Selector35/1  "<normalizedScopeValues>"
  Data Type Conversion53/1 -> Byte Pack1/57
  Data Type Conversion54/1 -> Byte Pack1/58
  Bus Selector35/1 -> Data Type Conversion53/1  "<actual>"
  Bus Selector35/2 -> Data Type Conversion54/1  "<command>"
  Bus Selector36/2 -> Data Type Conversion56/1  "<command>"
  Bus Selector36/1 -> Data Type Conversion55/1  "<actual>"
  Bus Selector26/3 -> Bus Selector36/1  "<displayValues>"
  Data Type Conversion55/1 -> Byte Pack1/59
  Data Type Conversion56/1 -> Byte Pack1/60
  Data Type Conversion51/1 -> Byte Pack1/55
  Data Type Conversion50/1 -> Byte Pack1/54
  Bus Selector23/3 -> Bus Selector33/1  "<displayValues>"
  Bus Selector33/1 -> Data Type Conversion50/1  "<actual>"
  Bus Selector33/2 -> Data Type Conversion51/1  "<command>"
  Bus Selector32/2 -> Data Type Conversion49/1  "<command>"
  Bus Selector32/1 -> Data Type Conversion48/1  "<actual>"
  Data Type Conversion49/1 -> Byte Pack1/53
  Data Type Conversion48/1 -> Byte Pack1/52
  Bus Selector23/2 -> Bus Selector32/1  "<normalizedScopeValues>"
  Bus Selector23/1 -> Data Type Conversion47/1  "<asciiLabel>"
  Data Type Conversion47/1 -> Byte Pack1/51
  Bus Selector14/1 -> Bus Selector3/1  "<actuatorPlot>"
  Bus Selector3/5 -> Bus Selector23/1  "<actuator5>"
  Bus Selector3/4 -> Bus Selector22/1  "<actuator4>"
  Bus Selector3/6 -> Bus Selector26/1  "<actuator6>"
  Bus Selector3/3 -> Bus Selector19/1  "<actuator3>"
  Bus Selector3/7 -> Bus Selector29/1  "<actuator7>"
  Bus Selector3/2 -> Bus Selector15/1  "<actuator2>"
  Bus Selector3/8 -> Bus Selector30/1  "<actuator8>"
  Bus Selector3/1 -> Bus Selector16/1  "<actuator1>"
  Data Type Conversion67/1 -> Byte Pack1/3

== system RCD2/To RCD2/RCD2 Command Unpack ==
  bytes : Inport  OutDataTypeStr=uint8
  length : Inport  Port=2  OutDataTypeStr=int32  PortDimensions=1
  AND : Logic  AllPortsSameDT=off  OutDataTypeStr=boolean
  AND1 : Logic  AllPortsSameDT=off  OutDataTypeStr=boolean
  Check Message Size : simulink/Logic and Bit Operations/Compare To Constant  relop===  const=int32(323)  OutDataTypeStr=boolean
  Relational Operator : RelationalOperator  Operator=<=  OutDataTypeStr=boolean  RndMeth=Simplest  InputSameDT=off
  Unpack Message : Subsystem  TreatAsAtomicUnit=on
  Width : Width  DataType=int32
  success : Outport
  rcd2Command : Outport  Port=2
  wires:
  bytes/1 -> Width/1, Unpack Message/1(bytes)
  AND1/1 -> Unpack Message/Enable, AND/1
  AND/1 -> success/1
  length/1 -> Relational Operator/1, Check Message Size/1
  Unpack Message/1(success) -> AND/2
  Unpack Message/2(busRCDCommand) -> rcd2Command/1
  Check Message Size/1 -> AND1/1
  Relational Operator/1 -> AND1/2
  Width/1 -> Relational Operator/2

== system RCD2/From RCD2/RCD2 Actual Pack/LED to uint16 ==
  "LED " : Inport
  Bitwise AND5 : simulink/Logic and Bit Operations/Bitwise Operator  logicop=OR  UseBitMask=off  NumInputPorts=8  BitMask=bin2dec('11011001')  BitMaskRealWorld=Stored Integer
      settings: LibrarySourceBlock=|
      | simulink/Quick Insert/Logic and Bit
      | Operations/Bitwise AND
  Bus Selector : BusSelector  OutputSignals=LED1,LED2,LED3,LED4,LED5,LED6,LED7,LED8  OutputAsBus=on
  Bus to Vector : BusToVector
  Data Type Conversion : DataTypeConversion  OutDataTypeStr=uint16  SaturateOnIntegerOverflow=off  RndMeth=Floor
  Demux1 : Demux  Outputs=8
  Saturation : Saturate  UpperLimit=uint8(3)  LowerLimit=uint8(0)
  Shift Arithmetic10 : ArithShift  BitShiftNumber=12  BitShiftDirection=Left
  Shift Arithmetic11 : ArithShift  BitShiftNumber=14  BitShiftDirection=Left
  Shift Arithmetic12 : ArithShift  BitShiftNumber=8  BitShiftDirection=Left
  Shift Arithmetic3 : ArithShift  BitShiftNumber=2  BitShiftDirection=Left
  Shift Arithmetic7 : ArithShift  BitShiftNumber=4  BitShiftDirection=Left
  Shift Arithmetic8 : ArithShift  BitShiftNumber=6  BitShiftDirection=Left
  Shift Arithmetic9 : ArithShift  BitShiftNumber=10  BitShiftDirection=Left
  u16 : Outport
  wires:
  Shift Arithmetic8/1 -> Bitwise AND5/4
  Demux1/4 -> Shift Arithmetic8/1
  Demux1/2 -> Shift Arithmetic3/1
  Demux1/3 -> Shift Arithmetic7/1
  Demux1/7 -> Shift Arithmetic10/1
  Shift Arithmetic7/1 -> Bitwise AND5/3
  Shift Arithmetic12/1 -> Bitwise AND5/5
  Demux1/8 -> Shift Arithmetic11/1
  Shift Arithmetic3/1 -> Bitwise AND5/2
  Shift Arithmetic9/1 -> Bitwise AND5/6
  Demux1/1 -> Bitwise AND5/1
  Shift Arithmetic10/1 -> Bitwise AND5/7
  Shift Arithmetic11/1 -> Bitwise AND5/8
  Demux1/5 -> Shift Arithmetic12/1
  Demux1/6 -> Shift Arithmetic9/1
  Bitwise AND5/1 -> u16/1
  "LED "/1 -> Bus Selector/1
  Bus Selector/1 -> Bus to Vector/1
  Bus to Vector/1 -> Saturation/1
  Data Type Conversion/1 -> Demux1/1
  Saturation/1 -> Data Type Conversion/1

== system RCD2/From RCD2/RCD2 Actual Pack/taster to uint16 ==
  "taster " : Inport
  Bitwise AND5 : simulink/Logic and Bit Operations/Bitwise Operator  logicop=OR  UseBitMask=off  NumInputPorts=16  BitMask=bin2dec('11011001')  BitMaskRealWorld=Stored Integer
      settings: LibrarySourceBlock=|
      | simulink/Quick Insert/Logic and Bit
      | Operations/Bitwise AND
  Bus Selector : BusSelector  OutputSignals=taster1,taster2,taster3,taster4,taster5,taster6,taster7,taster8,taster9,taster10,taster11,taster12,taster13,taster14,taster15,taster16  OutputAsBus=on
  Bus to Vector : BusToVector
  Data Type Conversion : DataTypeConversion  OutDataTypeStr=uint16  SaturateOnIntegerOverflow=off  RndMeth=Floor
  Demux1 : Demux  Outputs=16
  Shift Arithmetic1 : ArithShift  BitShiftNumber=1  BitShiftDirection=Left
  Shift Arithmetic10 : ArithShift  BitShiftNumber=12  BitShiftDirection=Left
  Shift Arithmetic11 : ArithShift  BitShiftNumber=14  BitShiftDirection=Left
  Shift Arithmetic12 : ArithShift  BitShiftNumber=8  BitShiftDirection=Left
  Shift Arithmetic13 : ArithShift  BitShiftNumber=11  BitShiftDirection=Left
  Shift Arithmetic14 : ArithShift  BitShiftNumber=13  BitShiftDirection=Left
  Shift Arithmetic15 : ArithShift  BitShiftNumber=15  BitShiftDirection=Left
  Shift Arithmetic2 : ArithShift  BitShiftNumber=3  BitShiftDirection=Left
  Shift Arithmetic3 : ArithShift  BitShiftNumber=2  BitShiftDirection=Left
  Shift Arithmetic4 : ArithShift  BitShiftNumber=5  BitShiftDirection=Left
  Shift Arithmetic5 : ArithShift  BitShiftNumber=7  BitShiftDirection=Left
  Shift Arithmetic6 : ArithShift  BitShiftNumber=9  BitShiftDirection=Left
  Shift Arithmetic7 : ArithShift  BitShiftNumber=4  BitShiftDirection=Left
  Shift Arithmetic8 : ArithShift  BitShiftNumber=6  BitShiftDirection=Left
  Shift Arithmetic9 : ArithShift  BitShiftNumber=10  BitShiftDirection=Left
  u16 : Outport
  wires:
  Data Type Conversion/1 -> Demux1/1
  Bus Selector/1 -> Bus to Vector/1
  "taster "/1 -> Bus Selector/1
  Bitwise AND5/1 -> u16/1
  Demux1/6 -> Shift Arithmetic4/1
  Demux1/5 -> Shift Arithmetic7/1
  Shift Arithmetic5/1 -> Bitwise AND5/8
  Shift Arithmetic8/1 -> Bitwise AND5/7
  Demux1/1 -> Bitwise AND5/1
  Shift Arithmetic4/1 -> Bitwise AND5/6
  Shift Arithmetic1/1 -> Bitwise AND5/2
  Demux1/8 -> Shift Arithmetic5/1
  Shift Arithmetic7/1 -> Bitwise AND5/5
  Shift Arithmetic3/1 -> Bitwise AND5/3
  Demux1/7 -> Shift Arithmetic8/1
  Demux1/3 -> Shift Arithmetic3/1
  Demux1/2 -> Shift Arithmetic1/1
  Demux1/4 -> Shift Arithmetic2/1
  Shift Arithmetic2/1 -> Bitwise AND5/4
  Bus to Vector/1 -> Data Type Conversion/1
  Demux1/9 -> Shift Arithmetic12/1
  Demux1/10 -> Shift Arithmetic6/1
  Demux1/11 -> Shift Arithmetic9/1
  Demux1/12 -> Shift Arithmetic13/1
  Demux1/13 -> Shift Arithmetic10/1
  Demux1/14 -> Shift Arithmetic14/1
  Demux1/15 -> Shift Arithmetic11/1
  Demux1/16 -> Shift Arithmetic15/1
  Shift Arithmetic12/1 -> Bitwise AND5/9
  Shift Arithmetic6/1 -> Bitwise AND5/10
  Shift Arithmetic9/1 -> Bitwise AND5/11
  Shift Arithmetic13/1 -> Bitwise AND5/12
  Shift Arithmetic10/1 -> Bitwise AND5/13
  Shift Arithmetic14/1 -> Bitwise AND5/14
  Shift Arithmetic11/1 -> Bitwise AND5/15
  Shift Arithmetic15/1 -> Bitwise AND5/16
